simulink model "mobile_inverted_pendulum_v2"  (R2017b)
settings: Solver=ode23  StartTime=0.0  StopTime=50  MaxStep=80.0  RelTol=1e-3
libraries: simulink x1
settings Model: Creator=ANANDA RANGAN N  LastModifiedBy=ANANDA RANGAN N

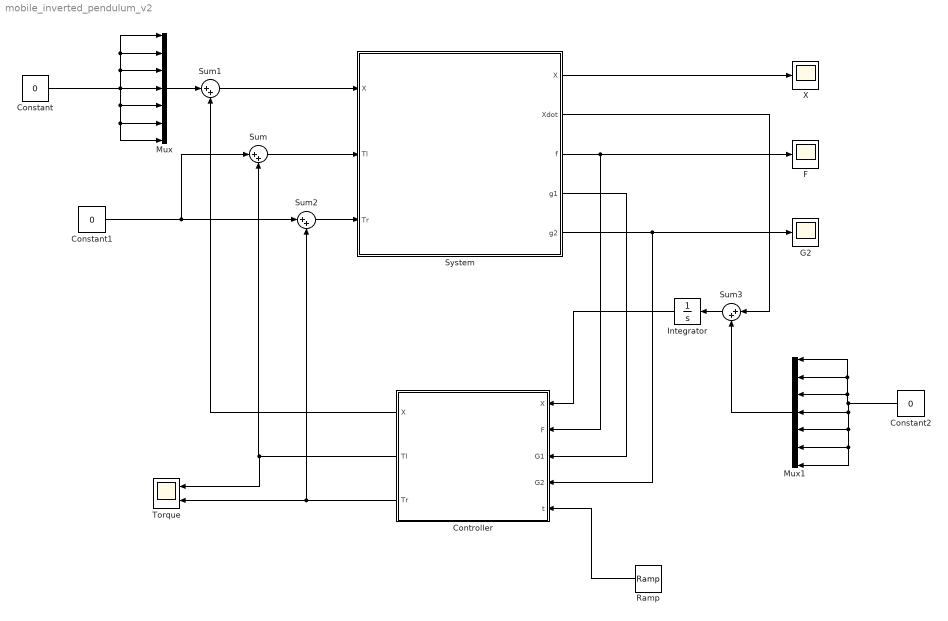
== system mobile_inverted_pendulum_v2 ==
  Constant : Constant  Value=0
  Constant1 : Constant  Value=0
  Constant2 : Constant  Value=0
  Controller : MATLAB Function  TreatAsAtomicUnit=on
  F : Scope
  G2 : Scope
  Integrator : Integrator
  Mux : Mux  Inputs=7
  Mux1 : Mux  Inputs=7
  Ramp : simulink/Sources/Ramp  slope=1  start=0  X0=0
  Sum{,1..3} (4 alike) : Sum  Inputs=|++
  System : MATLAB Function  TreatAsAtomicUnit=on
  Torque : Scope  NumInputPorts=2
  X : Scope
  wires:
  Mux/1 -> Sum1/1
  System/2(Xdot) -> Sum3/1
  System/3(f) -> Controller/2(F), F/1
  System/4(g1) -> Controller/3(G1)
  System/5(g2) -> Controller/4(G2), G2/1
  Integrator/1 -> Controller/1("X ")
  Sum1/1 -> System/1("X ")
  Constant/1 -> Mux/7, Mux/6, Mux/5, Mux/4, Mux/3, Mux/2, Mux/1
  Sum/1 -> System/2(Tl)
  Sum2/1 -> System/3(Tr)
  Controller/2(Tl) -> Torque/1, Sum/2
  Controller/3(Tr) -> Torque/2, Sum2/2
  Constant1/1 -> Sum2/1, Sum/1
  System/1(X) -> X/1
  Constant2/1 -> Mux1/4, Mux1/5, Mux1/6, Mux1/7, Mux1/3, Mux1/2, Mux1/1
  Sum3/1 -> Integrator/1
  Mux1/1 -> Sum3/2
  Controller/1(X) -> Sum1/2
  Ramp/1 -> Controller/5(t)

== matlab function mobile_inverted_pendulum_v2/Controller ==
  data: X output; X input; Tl output; F input; G1 input; G2 input; Tr output; t input
function [X, Tl, Tr] = fcn(X, F, G1, G2, t)

Tl = 0;
Tr = 0;
x = X(1); y = X(2); theta = X(3); a = X(4);
adot = X(5); v = X(6); tdot = X(7);

%control algorithm

x_desired = 0.2; y_desired = -0.4; theta_desired = 0.6; k = 0.0001;

if k > abs(x - x_desired)
    k = abs(x - x_desired);
end

if y_desired == 0;
% push the pendulum out of equilibrium if the bot is at rest and not at the desired location
%
    if (x > x_desired+0.001) || (x < x_desired-0.001) 
%        if (v <0.1) && (v>-0.1)                               
%            if (a<0.01) && (a>-0.01)                            
                if x < x_desired - 0.005
                    X(4) = -k;     %   a = -0.1
                else if x > x_desired + 0.005
                    X(4) = k;    %   a = 0.1
                    end
                end
%            end
%        end

    Kp = 5; Kd = 1; Kd_x = -1;

    Tl = Kp*(a-0) + Kd*(adot-0) + Kd_x*(v - 0);
    Tr = Kp*(a-0) + Kd*(adot-0) + Kd_x*(v - 0);
    end
end
%
if x_desired == 0
    theta_initial = (pi)/2;
else 
    theta_initial = y_desired/x_desired;
end
    if ((tan(theta) < theta_initial-0.001) || (tan(theta) > theta_initial+0.001) || (tdot>0.01) || (tdot<-0.01)) && t<100
        Kp = 5; Kd = 10;
        Tl = Kp*(tan(theta) - theta_initial) + Kd*(tdot - 0);
        Tr = -Tl;

        
    k = 0.0001;
    if k > abs(x - x_desired)
     k = abs(x - x_desired);
    end

    else if ((x > x_desired+0.001) || (x < x_desired-0.001))
%        if (v <0.1) && (v>-0.1)                               
%            if (a<0.01) && (a>-0.01)                            
                if x < x_desired - 0.005
                    X(4) = -0.00925;     %   a = -0.1
                else if x > x_desired + 0.005
                    X(4) = 0.00925;    %   a = 0.1
                    end
                end
%            end
%        end

        Kp = 5; Kd = 1; Kd_x = -5; Kp_theta = 5; Kd_theta = 10;

        Tl = Kp*(a-0) + Kd*(adot-0) + Kd_x*(v - 0) + Kp_theta*(tan(theta) - theta_initial) + Kd_theta*(tdot - 0);
        Tr = Kp*(a-0) + Kd*(adot-0) + Kd_x*(v - 0) - Kp_theta*(tan(theta) - theta_initial) - Kd_theta*(tdot - 0);  
      end
    end
    
if t>20
   Kp = 15; Kd = 1; Kd_x = -5; Kp_theta = 5; Kd_theta = 10;

    Tl = Kp*(a-0) + Kd*(adot-0) + Kd_x*(v - 0) + Kp_theta*(theta - theta_desired) + Kd_theta*(tdot - 0);
    Tr = Kp*(a-0) + Kd*(adot-0) + Kd_x*(v - 0) - Kp_theta*(theta - theta_desired) - Kd_theta*(tdot - 0);  
end
%
%

== matlab function mobile_inverted_pendulum_v2/System ==
  data: X output; X input; Xdot output; Tl input; Tr input; f output; g1 output; g2 output
function [X, Xdot, f, g1, g2] = fcn(X, Tl, Tr)

%{
  x = ( x, y, theta, alpha, alpha_dot, v, theta_dot)
  Mb = mass of the bot
  Mw = ??
  cz = centre of mass along z direction
  Ix, Iy, Iz = Moment of Inertia along X, Y, Z axes
  Iwa = Moment of Inertia along wheel axis
  Iwd = ??
  R = Radius of the wheel
  b = distance between the wheels
%}
%system parameters
Mb = 3.9;  Mw = 0.375;
cz = 0.1;
Ix = 0.02; Iy = 0.015; Iz = 0.01;
Iwa = 0.001; Iwd = 0.002; 
R = 0.1025; b = 0.1620;
g = 9.81;

%matrix dimension declaration
f = [0;0;0;0;0;0;0]; g1 = f; g2 = g1; Xdot = f;

%variable declaration
if X(4) < -1.57
    X(4) = -1.57;
else if X(4) > 1.57
        X(4) = 1.57;
    end 
end 

x = X(1); y = X(2); theta = X(3); a = X(4);
adot = X(5); v = X(6); tdot = X(7);


%intermediate variables
b1 = (Mb*cz*cz) + Ix - Iz;
b2 = (Mb*cz*cz) + Iy;
b3 = ((Mb*R*R) + 2*(Iwa + (Mw*R*R)))/(R*R);
b4 = ((R*R)*(Iz + (2*Iwd) + (2*b*b*Mw)) + (2*b*b*Iwa))/(R*R);
b5 = Mb*cz;

T1 = (b2*b3) - (b5*b5*cos(a)*cos(a))     + 0.0000000001;
T2 = b4 + (b1*sin(a)*sin(a))     + 0.0000000001;

g5 = (b3*R) + (b5*cos(a));
g6 = b2 + (R*b5*cos(a));

denom = 2*((b2*b3) - (b5*b5*cos(a)*cos(a)))     + 0.0000000001;


f(1) = v*(cos(theta));
f(2) = v*(sin(theta));
f(3) = tdot;
f(4) = adot;
f(5) = (sin(2*a)*((b3*b1*tdot*tdot)-(b5*b5*adot*adot)) + (2*b5*b3*sin(a)))/denom;
f(6) = ((2*b2*b5*adot*adot*sin(a)) - sin(2*a)*((b1*b5*tdot*tdot*cos(a)) + (b5*b5*g)))/denom;
f(7) = (-b1*adot*tdot*sin(2*a))/(b4 + (b1*sin(a)*sin(a))   + 0.000000000001);


g1(1) = 0; g1(2) = 0; g1(3) = 0; g1(4) = 0;
g1(5) = -g5/(R*T1);
g1(6) = g6/(R*T1);
g1(7) = b/(R*T2);

g2(1) = 0; g2(2) = 0; g2(3) = 0; g2(4) = 0;
g2(5) = -g5/(R*T1);
g2(6) = g6/(R*T1);
g2(7) = -b/(R*T2);


Xdot = f + (g1.*Tr) + (g2.*Tl);
